simulink library "Storage_Type_3"  (Simulink 8.2)
settings: Solver=ode45  StartTime=0.0  StopTime=10.0  RelTol=1e-3
libraries: carnot x8
settings Model: Creator=lena.frank  LastModifiedBy=drhf

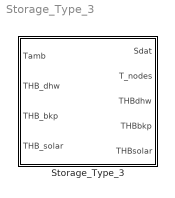
== system Storage_Type_3 ==
  Storage_Type_3 : Subsystem  mask(Multiport Storage){uloss=1, ubot=1, utop=1, cond=1, t0=[10:5:55], volume=0.3, dia=0.5, pos=standing cylinder, nconnect=3, nodes=10, mpoints=10}
      mask prompts: uloss "Heat loss coefficient cylinder wall in W/(m²K)"; ubot "Heat loss coefficient bottom in W/(m²K)"; utop "Heat loss coefficient top cover in W/(m²K)"; cond "Effective (wall and fluid) vertical conductivity in W/(m*K)"; t0 "Initial temperature (vector or scalar) in °C"; volume "Volume in m³"; dia "Diameter in m"; pos "Position"; nconnect "Number of connections"; nodes "Number of nodes"; mpoints "Number of measurement points"
      mask help:
      | The volmue of the cylindrical storage is divided in a number "nodes" of horizontal slices (1xN-node model). For each node the energy balance equation is solved.
      | Look under mask to set the ports types and properties.
      mask init:
      | [standing, dh, height, mpts, tini] ...
      |     = CarnotCallbacks_StorageTypeN(pos, volume, dia, nodes, mpoints, t0);
      mask Help: web(fullfile(path_carnot('help'),'Storage_Type_N.html'),'-helpbrowser')
      mask TypeOptions pos: lying cylinder | standing cylinder
      mask Display: plot(10,20,80,100,[36,36,40,50,54,54,50,40,36],[90,50,45,45,50,90,93,93,90],[36,51,40,51,36],[77,77,81,85,85],[36,51,44,51,36],[50,50,55,60,60])

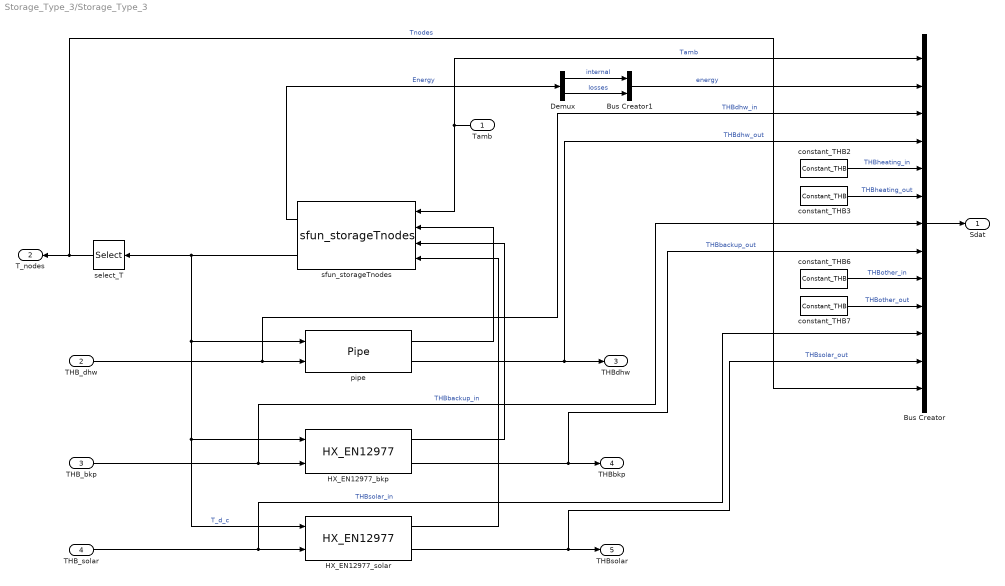
== system Storage_Type_3/Storage_Type_3 ==
  Tamb : Inport
  THB_dhw : Inport  Port=2
  THB_bkp : Inport  Port=3
  THB_solar : Inport  Port=4
  Bus Creator : BusCreator  Inputs=13
  Bus Creator1 : BusCreator  Inputs=2
  Demux : Demux  Outputs=2
  HX_EN12977_bkp : carnot/Storage/Thermal/Storage_Ports/HX_EN12977  h_in=0.81  h_out=0.56  ua0=80  uam=0.2  uat=0.5  dplin=100  dpqua=100  nodes=nodes  hgt=height  dia=dia
  HX_EN12977_solar : carnot/Storage/Thermal/Storage_Ports/HX_EN12977  h_in=0.48  h_out=0.04  ua0=100  uam=0.2  uat=0.5  dplin=100  dpqua=100  nodes=nodes  hgt=height  dia=dia
  constant_THB{2..3,6..7} (4 alike) : carnot/Source/Simple/Constant_THB  t=20  mdot=0  p=1e5  mID=No Pressure Drop  fluid=Water  mix=0  dia=0.02  hgt=0
  pipe : carnot/Storage/Thermal/Storage_Ports/Pipe  h_in=0  h_out=1  dplin=10  dpqua=10  nodes=nodes  hgt=height  dia=dia
  select_T : Selector  InputPortWidth=nodes  IndexOptions=Index vector (dialog)  Indices=mpts  OutputSizes=1
  sfun_storageTnodes : carnot/Basic/Thermal_Models/sfun_storageTnodes  dia=dia  volume=volume  standing=standing  uloss=uloss  ubot=utop  utop=ubot  cond=cond  tini=tini  nodes=nodes  nconnect=nconnect
  Sdat : Outport
  T_nodes : Outport  Port=2
  THBdhw : Outport  Port=3
  THBbkp : Outport  Port=4
  THBsolar : Outport  Port=5
  wires:
  HX_EN12977_solar/2 -> Bus Creator/12, THBsolar/1  "THBsolar_out"
  THB_solar/1 -> Bus Creator/11, HX_EN12977_solar/2  "THBsolar_in"
  HX_EN12977_solar/1 -> sfun_storageTnodes/4
  Bus Creator1/1 -> Bus Creator/2  "energy"
  Demux/2 -> Bus Creator1/2  "losses"
  Demux/1 -> Bus Creator1/1  "internal"
  HX_EN12977_bkp/1 -> sfun_storageTnodes/3
  HX_EN12977_bkp/2 -> Bus Creator/8, THBbkp/1  "THBbackup_out"
  THB_bkp/1 -> Bus Creator/7, HX_EN12977_bkp/2  "THBbackup_in"
  constant_THB3/1 -> Bus Creator/6  "THBheating_out"
  constant_THB2/1 -> Bus Creator/5  "THBheating_in"
  constant_THB6/1 -> Bus Creator/9  "THBother_in"
  constant_THB7/1 -> Bus Creator/10  "THBother_out"
  Bus Creator/1 -> Sdat/1
  sfun_storageTnodes/2 -> HX_EN12977_solar/1, HX_EN12977_bkp/1, pipe/1, select_T/1  "T_d_c"
  sfun_storageTnodes/1 -> Demux/1  "Energy"
  select_T/1 -> Bus Creator/13, T_nodes/1  "Tnodes"
  pipe/1 -> sfun_storageTnodes/2
  pipe/2 -> Bus Creator/4, THBdhw/1  "THBdhw_out"
  THB_dhw/1 -> Bus Creator/3, pipe/2  "THBdhw_in"
  Tamb/1 -> Bus Creator/1, sfun_storageTnodes/1  "Tamb"
